simulink subsystem "rss_GDVltgCalc"  (R2023a)
settings: Solver=VariableStepAuto  StartTime=0.0  StopTime=10.0  RelTol=1e-3
undefined symbols (not defined in the file): Cdbl_uCtlBrdVltgPeakVal, Gu16_rGDVltgADCRat_C
libraries: lib_conversion x2, lib_moving_average_filter x1
settings Model: Creator=xiaoqiang.yuan  LastModifiedBy=xiaoqiang.yuan

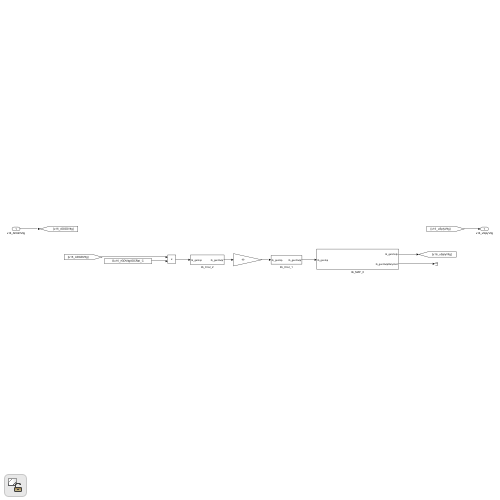
[thumbnail: Simulink's stored preview of the top-level diagram]
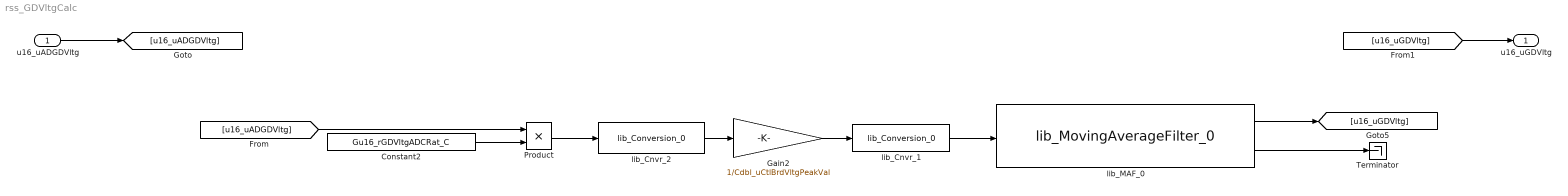
== system rss_GDVltgCalc ==
  u16_uADGDVltg : Inport  OutDataTypeStr=uint16
  Constant2 : Constant  Value=Gu16_rGDVltgADCRat_C
  Gain2 : Gain  Gain=1/Cdbl_uCtlBrdVltgPeakVal  OutDataTypeStr=Inherit: Inherit via back propagation
  Product : Product  OutDataTypeStr=Inherit: Inherit via back propagation
  Terminator : Terminator
  lib_Cnvr_1 : lib_conversion/lib_Conversion_0  lb_parDataType=dt_Standardize_u16p15b0  lb_parOutpMaxVal=[]  lb_parOutpMinVal=[]  lb_parSatFlag=off
  lib_Cnvr_2 : lib_conversion/lib_Conversion_0  lb_parDataType=fixdt(1,16)  lb_parOutpMaxVal=Cdbl_uCtlBrdVltgPeakVal  lb_parOutpMinVal=[]  RndMeth=Simplest  lb_parSatFlag=off
  lib_MAF_0 : lib_moving_average_filter/lib_MovingAverageFilter_0  lb_parSampNum=Cdbl_numGDVltgMAFSmpNum  lb_parInpSmtnDataType=fixdt(1,32,2^-19,0)
  u16_uGDVltg : Outport  OutDataTypeStr=dt_Standardize_u16p15b0
  wires:
  lib_MAF_0/1 -> [u16_uGDVltg]
  [u16_uADGDVltg] -> Product/1
  Constant2/1 -> Product/2
  Product/1 -> lib_Cnvr_2/1
  lib_Cnvr_1/1 -> lib_MAF_0/1
  lib_MAF_0/2 -> Terminator/1
  lib_Cnvr_2/1 -> Gain2/1
  Gain2/1 -> lib_Cnvr_1/1
  [u16_uGDVltg] -> u16_uGDVltg/1
  u16_uADGDVltg/1 -> [u16_uADGDVltg]
